simulink model "k1visetmyp"  (Simulink 8.6)
settings: Solver=ode45  StartTime=0.0  StopTime=10.0  RelTol=1e-3
libraries: cdsIPCx x50, cdsFilt x11, cdsCDI64 x6, cdsCDO64 x6, BIO_CD_DECODE_MASTER x6, BIO_CD_ENCODE_MASTER x5, CHK_DIO x5, dac x3, cdsBit2Word x2, cdsAdcx0 x1, cdsAdcx1 x1, TYPEA_MASTER x1
(part 2 of 2)

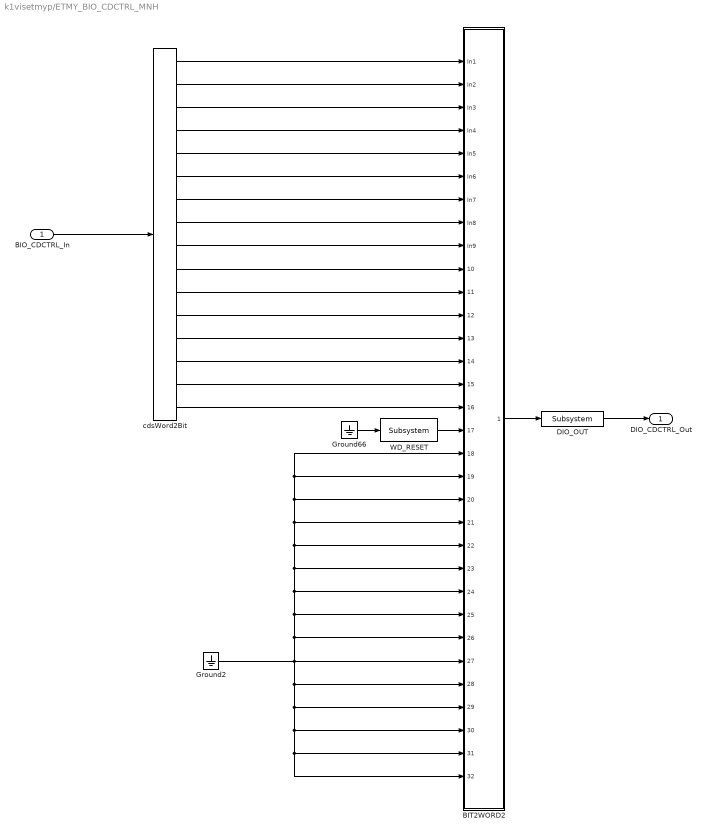
== system k1visetmyp/ETMY_BIO_CDCTRL_MNH ==
  BIO_CDCTRL_In : Inport
  BIT2WORD2 : Subsystem
  DIO_OUT : cdsEpicsOut/Subsystem  Tag=cdsEpicsOutput  Description=|
      | Purpose:                                          
      | Output a FE signal to an EPICS channel.           
      |                                                   
      | Operation:                                        
      | Takes input value and passes it to EPICS record.  
      |                                                   
      | Usage:                                            
      | Name the part with the desired EPICS rrecord name.
      settings: AttributesFormatString=%<Tag>
  Ground2 : Ground
  Ground66 : Ground
  WD_RESET : cdsEpicsBinIn/Subsystem  Tag=cdsEpicsBinIn  Description=|
      | Purpose:                                                                            
      | Create an EPICS binary (0 or 1) input channel to the FE realtime controls.          
      |                                                                                     
      | Operation:                                                                          
      | Outputs value from an EPICS ai record. Value is binary input (bi Epics record type).
      |                                                                                     
      | Usage:                                                                              
      | Name the part with the desired EPICS channel name.
      settings: AttributesFormatString=%<Tag>
  cdsWord2Bit : cdsWord2Bit/cdsWord2Bit  Tag=cdsWord2Bit  Description=Generate 16 0/1 outputs from single 16-bit integer input
      settings: AttributesFormatString=cdsWord2Bit
  DIO_CDCTRL_Out : Outport
  wires:
  BIT2WORD2/1(Out1) -> DIO_OUT/1
  DIO_OUT/1 -> DIO_CDCTRL_Out/1
  BIO_CDCTRL_In/1 -> cdsWord2Bit/1
  cdsWord2Bit/1 -> BIT2WORD2/1(In1)
  cdsWord2Bit/2 -> BIT2WORD2/2(In2)
  cdsWord2Bit/3 -> BIT2WORD2/3(In3)
  cdsWord2Bit/4 -> BIT2WORD2/4(In4)
  cdsWord2Bit/5 -> BIT2WORD2/5(In5)
  cdsWord2Bit/6 -> BIT2WORD2/6(In6)
  cdsWord2Bit/7 -> BIT2WORD2/7(In7)
  cdsWord2Bit/8 -> BIT2WORD2/8(In8)
  cdsWord2Bit/9 -> BIT2WORD2/9(In9)
  cdsWord2Bit/10 -> BIT2WORD2/10(In10)
  cdsWord2Bit/11 -> BIT2WORD2/11(In11)
  cdsWord2Bit/12 -> BIT2WORD2/12(In12)
  cdsWord2Bit/13 -> BIT2WORD2/13(In13)
  cdsWord2Bit/14 -> BIT2WORD2/14(In14)
  cdsWord2Bit/15 -> BIT2WORD2/15(In15)
  cdsWord2Bit/16 -> BIT2WORD2/16(In16)
  WD_RESET/1 -> BIT2WORD2/17(In17)
  Ground66/1 -> WD_RESET/1
  Ground2/1 -> BIT2WORD2/27(In27), BIT2WORD2/28(In28), BIT2WORD2/29(In29), BIT2WORD2/30(In30), BIT2WORD2/31(In31), BIT2WORD2/32(In32), BIT2WORD2/26(In26), BIT2WORD2/25(In25), BIT2WORD2/24(In24), BIT2WORD2/23(In23), BIT2WORD2/22(In22), BIT2WORD2/21(In21), BIT2WORD2/20(In20), BIT2WORD2/18(In18), BIT2WORD2/19(In19)

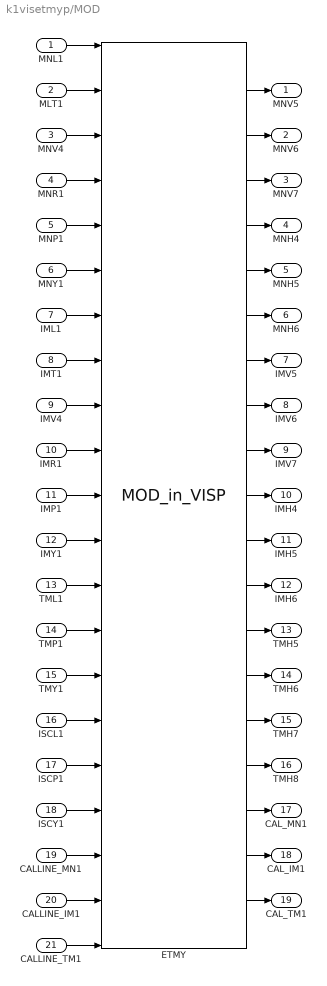
== system k1visetmyp/MOD ==
  MNL1 : Inport
  MLT1 : Inport  Port=2
  MNV4 : Inport  Port=3
  MNR1 : Inport  Port=4
  MNP1 : Inport  Port=5
  MNY1 : Inport  Port=6
  IML1 : Inport  Port=7
  IMT1 : Inport  Port=8
  IMV4 : Inport  Port=9
  IMR1 : Inport  Port=10
  IMP1 : Inport  Port=11
  IMY1 : Inport  Port=12
  TML1 : Inport  Port=13
  TMP1 : Inport  Port=14
  TMY1 : Inport  Port=15
  ISCL1 : Inport  Port=16
  ISCP1 : Inport  Port=17
  ISCY1 : Inport  Port=18
  CALLINE_MN1 : Inport  Port=19
  CALLINE_IM1 : Inport  Port=20
  CALLINE_TM1 : Inport  Port=21
  ETMY : VIS_LIB/MODAL/MOD_in_VISP  Tag=top_names
  MNV5 : Outport
  MNV6 : Outport  Port=2
  MNV7 : Outport  Port=3
  MNH4 : Outport  Port=4
  MNH5 : Outport  Port=5
  MNH6 : Outport  Port=6
  IMV5 : Outport  Port=7
  IMV6 : Outport  Port=8
  IMV7 : Outport  Port=9
  IMH4 : Outport  Port=10
  IMH5 : Outport  Port=11
  IMH6 : Outport  Port=12
  TMH5 : Outport  Port=13
  TMH6 : Outport  Port=14
  TMH7 : Outport  Port=15
  TMH8 : Outport  Port=16
  CAL_MN1 : Outport  Port=17
  CAL_IM1 : Outport  Port=18
  CAL_TM1 : Outport  Port=19
  wires:
  MNL1/1 -> ETMY/1
  TMY1/1 -> ETMY/15
  MLT1/1 -> ETMY/2
  MNV4/1 -> ETMY/3
  MNR1/1 -> ETMY/4
  MNP1/1 -> ETMY/5
  MNY1/1 -> ETMY/6
  IML1/1 -> ETMY/7
  IMT1/1 -> ETMY/8
  IMV4/1 -> ETMY/9
  IMR1/1 -> ETMY/10
  IMP1/1 -> ETMY/11
  IMY1/1 -> ETMY/12
  TML1/1 -> ETMY/13
  TMP1/1 -> ETMY/14
  ETMY/1 -> MNV5/1
  ETMY/16 -> TMH8/1
  ETMY/2 -> MNV6/1
  ETMY/3 -> MNV7/1
  ETMY/4 -> MNH4/1
  ETMY/5 -> MNH5/1
  ETMY/6 -> MNH6/1
  ETMY/7 -> IMV5/1
  ETMY/8 -> IMV6/1
  ETMY/9 -> IMV7/1
  ETMY/10 -> IMH4/1
  ETMY/11 -> IMH5/1
  ETMY/12 -> IMH6/1
  ETMY/13 -> TMH5/1
  ETMY/14 -> TMH6/1
  ETMY/15 -> TMH7/1
  ISCL1/1 -> ETMY/16
  CALLINE_TM1/1 -> ETMY/21
  CALLINE_IM1/1 -> ETMY/20
  CALLINE_MN1/1 -> ETMY/19
  ISCP1/1 -> ETMY/17
  ISCY1/1 -> ETMY/18
  ETMY/17 -> CAL_MN1/1
  ETMY/18 -> CAL_IM1/1
  ETMY/19 -> CAL_TM1/1

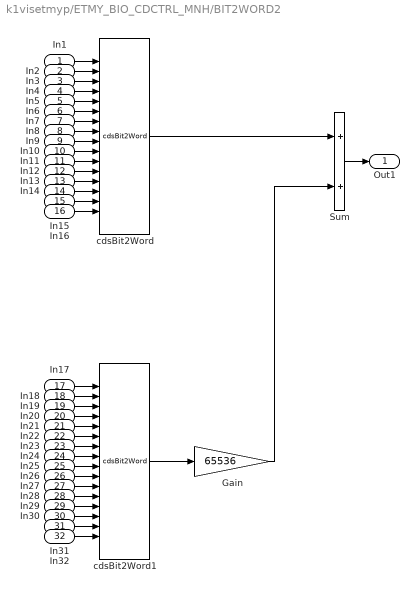
== system k1visetmyp/ETMY_BIO_CDCTRL_MNH/BIT2WORD2 ==
  In1 : Inport
  In2 : Inport  Port=2
  In3 : Inport  Port=3
  In4 : Inport  Port=4
  In5 : Inport  Port=5
  In6 : Inport  Port=6
  In7 : Inport  Port=7
  In8 : Inport  Port=8
  In9 : Inport  Port=9
  In10 : Inport  Port=10
  In11 : Inport  Port=11
  In12 : Inport  Port=12
  In13 : Inport  Port=13
  In14 : Inport  Port=14
  In15 : Inport  Port=15
  In16 : Inport  Port=16
  In17 : Inport  Port=17
  In18 : Inport  Port=18
  In19 : Inport  Port=19
  In20 : Inport  Port=20
  In21 : Inport  Port=21
  In22 : Inport  Port=22
  In23 : Inport  Port=23
  In24 : Inport  Port=24
  In25 : Inport  Port=25
  In26 : Inport  Port=26
  In27 : Inport  Port=27
  In28 : Inport  Port=28
  In29 : Inport  Port=29
  In30 : Inport  Port=30
  In31 : Inport  Port=31
  In32 : Inport  Port=32
  Gain : Gain  Gain=65536
  Sum : Sum
  cdsBit2Word : cdsBit2Word/cdsBit2Word  Tag=cdsBit2Word  Description=Forms single 16 bit integer from 16 0/1 inputs.
      settings: AttributesFormatString=%<Tag>
  cdsBit2Word1 : cdsBit2Word/cdsBit2Word  Tag=cdsBit2Word  Description=Forms single 16 bit integer from 16 0/1 inputs.
      settings: AttributesFormatString=%<Tag>
  Out1 : Outport
  wires:
  In32/1 -> cdsBit2Word1/16
  In31/1 -> cdsBit2Word1/15
  In30/1 -> cdsBit2Word1/14
  In29/1 -> cdsBit2Word1/13
  In28/1 -> cdsBit2Word1/12
  In27/1 -> cdsBit2Word1/11
  In26/1 -> cdsBit2Word1/10
  In25/1 -> cdsBit2Word1/9
  In24/1 -> cdsBit2Word1/8
  In23/1 -> cdsBit2Word1/7
  In22/1 -> cdsBit2Word1/6
  In21/1 -> cdsBit2Word1/5
  In20/1 -> cdsBit2Word1/4
  In19/1 -> cdsBit2Word1/3
  In18/1 -> cdsBit2Word1/2
  In17/1 -> cdsBit2Word1/1
  In16/1 -> cdsBit2Word/16
  In15/1 -> cdsBit2Word/15
  In14/1 -> cdsBit2Word/14
  In13/1 -> cdsBit2Word/13
  In12/1 -> cdsBit2Word/12
  In11/1 -> cdsBit2Word/11
  Sum/1 -> Out1/1
  In10/1 -> cdsBit2Word/10
  In9/1 -> cdsBit2Word/9
  In8/1 -> cdsBit2Word/8
  In7/1 -> cdsBit2Word/7
  In6/1 -> cdsBit2Word/6
  In5/1 -> cdsBit2Word/5
  In4/1 -> cdsBit2Word/4
  In3/1 -> cdsBit2Word/3
  In2/1 -> cdsBit2Word/2
  In1/1 -> cdsBit2Word/1
  cdsBit2Word/1 -> Sum/1
  cdsBit2Word1/1 -> Gain/1
  Gain/1 -> Sum/2
